simulink model "mcp_smib_swing"  (R2025b)
settings: Solver=ode23t  StartTime=0.0  StopTime=5  MaxStep=0.005  RelTol=1e-3
values from neighbouring files (symbols this model uses):
  D0 = 3.0    (= 3)    [build_minimal_cvs_phasor.m]    (also in probe_sps_cvs_smib.m)
  M0 = 12.0    (= 12)    [build_minimal_cvs_phasor.m]
  Pm0 = 0.5    [probe_sps_cvs_smib.m]
undefined symbols (not defined in the file or in its folder): delta0, L_H_const, Pe_scale, Vbase_const, wn_const
libraries: spsGroundLib x2, spsACVoltageSourceLib x1, spsControlledVoltageSourceLib x1, spsCurrentMeasurementLib x1, spsSeriesRLCBranchLib x1, spsVoltageMeasurementLib x1, sps_lib x1
settings Model: Creator=27443  LastModifiedBy=27443

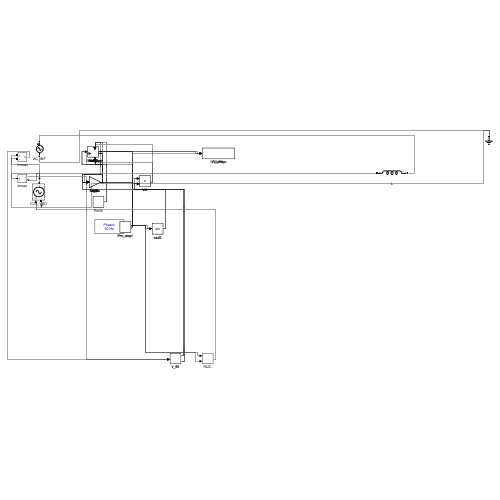
[thumbnail: Simulink's stored preview of the top-level diagram]
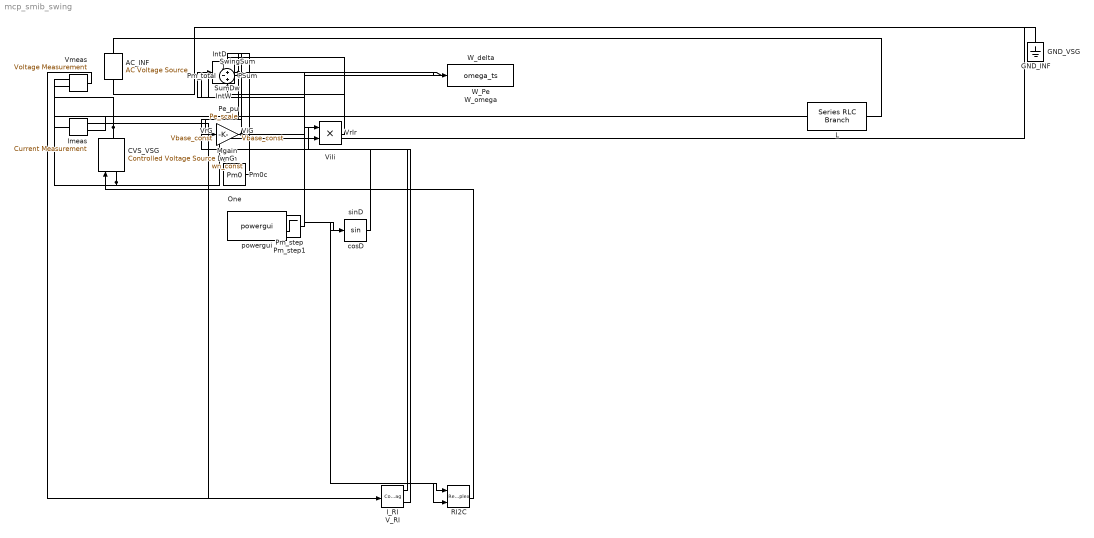
== system mcp_smib_swing ==
  AC_INF : spsACVoltageSourceLib/AC Voltage Source  Amplitude=230e3  Phase=0  Frequency=50  SampleTime=0  Measurements=None  BusType=swing  Pref=10e3  Qref=0  Qmin=-inf  Qmax=+inf
  CVS_VSG : spsControlledVoltageSourceLib/Controlled Voltage Source  Initialize=off  Source_Type=DC  Amplitude=230e3  Phase=0  Frequency=0  Measurements=None
  Dgain : Gain  Gain=D0
  GND_INF : spsGroundLib/Ground  LConnTagsString=a
  GND_VSG : spsGroundLib/Ground  LConnTagsString=a
  I_RI : ComplexToRealImag
  Imeas : spsCurrentMeasurementLib/Current Measurement  PhasorSimulation=on  OutputType=Complex  PSBequivalent=0
  IntD : Integrator  InitialCondition=delta0
  IntW : Integrator  InitialCondition=1
  L : spsSeriesRLCBranchLib/Series RLC Branch  LConnTagsString=__new0  RConnTagsString=__new0  BranchType=L  Resistance=1  Inductance=L_H_const  SetiL0=off  InitialCurrent=0  Capacitance=1e-6  Setx0=off  InitialVoltage=0  Measurements=None
  Mgain : Gain  Gain=1/M0
  One : Constant
  PSum : Sum
  Pe_pu : Gain  Gain=Pe_scale
  Pm0c : Constant  Value=Pm0
  Pm_step : Step  SampleTime=0
  Pm_step1 : Step  Time=2.0  After=0.1  SampleTime=0
  Pm_total : Sum
  RI2C : RealImagToComplex
  SumDw : Sum  Inputs=+-
  SwingSum : Sum  Inputs=+--
  V_RI : ComplexToRealImag
  ViG : Gain  Gain=Vbase_const
  ViIi : Product
  Vmeas : spsVoltageMeasurementLib/Voltage Measurement  PhasorSimulation=on  OutputType=Complex  PSBequivalent=0
  VrG : Gain  Gain=Vbase_const
  VrIr : Product
  W_Pe : ToWorkspace  VariableName=Pe_ts  SaveFormat=Timeseries  SampleTime=-1
  W_delta : ToWorkspace  VariableName=delta_ts  SaveFormat=Timeseries  SampleTime=-1
  W_omega : ToWorkspace  VariableName=omega_ts  SaveFormat=Timeseries  SampleTime=-1
  cosD : Trigonometry  Operator=cos
  powergui : sps_lib/powergui  Priority=1  SimulationMode=Phasor  SampleTime=50e-6  frequency=50  Iterations=50  frequencyindice=50  Pbase=100e6  ErrMax=1e-4  UnitsV=kV  UnitsW=MW  buscounter=0  FunctionMessages=off  echomessages=off  EnableUseOfTLC=off  CurrentSourceSwitches=off  DisableSnubberDevices=off  DisableRonSwitches=off  DisableVfSwitches=off  DisplayEquations=off  AutomaticDiscreteSolvers=off  SolverType=Tustin/Backward Euler (TBE)  Interpol=off  ExternalGateDelay=off  methode=off  Ts=100  x0status=blocks  SPID=on  SwTol=0  HookPort=off  NonlinearTolerance=1e-4  nMaxIteration=100  ContinueOnMaxIteration=off  RestoreLinks=warning  ResistiveCurrentMeasurement=off  Frange=[0:2:500]  Ylog=off  Xlog=on  ShowGrid=off  save=off  variable=ZData  structure=0  ZoomFFT=off  StartTime=0.0  cycles=1  DisplayStyle=1  fundamental=60  FreqAxis=off  MaxFrequency=1000  frequencyindicesteady=1  RmsSteady=1  display=off
  sinD : Trigonometry
  wnG : Gain  Gain=wn_const
  wires:
  Vmeas/1 -> V_RI/1
  Imeas/1 -> I_RI/1
  V_RI/1 -> VrIr/1
  I_RI/1 -> VrIr/2
  V_RI/2 -> ViIi/1
  I_RI/2 -> ViIi/2
  VrIr/1 -> PSum/1
  ViIi/1 -> PSum/2
  PSum/1 -> Pe_pu/1
  Pm0c/1 -> Pm_total/1
  Pm_step1/1 -> Pm_total/2
  IntW/1 -> SumDw/1, W_omega/1
  One/1 -> SumDw/2
  SumDw/1 -> Dgain/1, wnG/1
  Pm_total/1 -> SwingSum/1
  Pe_pu/1 -> SwingSum/2, W_Pe/1
  Dgain/1 -> SwingSum/3
  SwingSum/1 -> Mgain/1
  Mgain/1 -> IntW/1
  wnG/1 -> IntD/1
  IntD/1 -> cosD/1, sinD/1, W_delta/1
  cosD/1 -> VrG/1
  sinD/1 -> ViG/1
  VrG/1 -> RI2C/1
  ViG/1 -> RI2C/2
  RI2C/1 -> CVS_VSG/1
  connections:
  Imeas/LConn1 -- CVS_VSG/RConn1 -- Vmeas/LConn1
  Imeas/RConn1 -- L/LConn1
  GND_VSG/LConn1 -- CVS_VSG/LConn1 -- Vmeas/LConn2
  L/RConn1 -- AC_INF/RConn1
  AC_INF/LConn1 -- GND_INF/LConn1
